simulink model "Main2wheel_simulation"  (R2020b)
settings: Solver=ode4  StartTime=0.0  StopTime=5  FixedStep=0.00001  RelTol=1e-3
libraries: pid_lib x1
settings Model: Creator=Touch  LastModifiedBy=touch

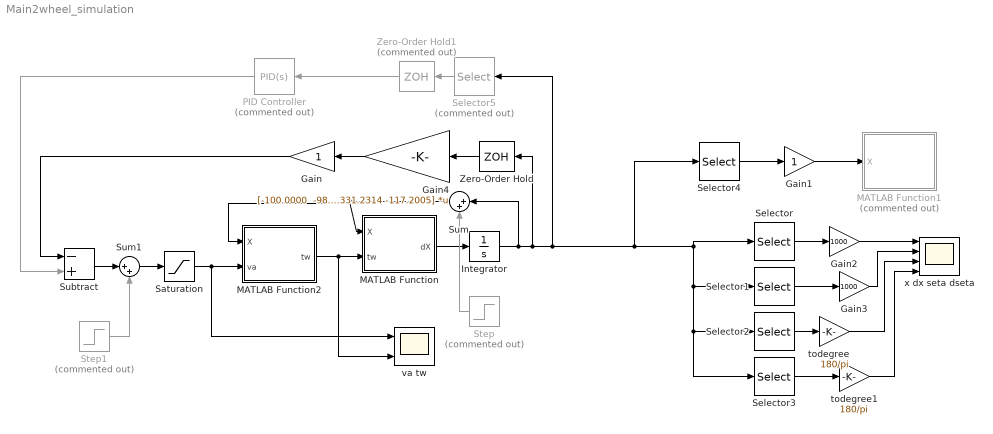
== system Main2wheel_simulation ==
  Gain : Gain
  Gain1 : Gain
  Gain2 : Gain  Gain=1000
  Gain3 : Gain  Gain=1000
  Gain4 : Gain  Gain="[-100.0000  -98.0599 -331.2314 -117.2005]"  Multiplication=Matrix(K*u)
  Integrator : Integrator  InitialCondition=[0;0;0.3;0]  UpperSaturationLimit=[inf;inf;pi/2;inf]  LowerSaturationLimit=[-inf;-inf;-pi/2;-inf]
  MATLAB Function : MATLAB Function  TreatAsAtomicUnit=on
  MATLAB Function1 : MATLAB Function  Commented=on  TreatAsAtomicUnit=on
  MATLAB Function2 : MATLAB Function  TreatAsAtomicUnit=on
  PID Controller : pid_lib/PID Controller  Commented=on  Controller=PID  Form=Parallel  TimeDomain=Continuous-time  UseExternalTs=off  SampleTime=-1  IntegratorMethod=Forward Euler  FilterMethod=Forward Euler  ControllerParametersSource=internal  P=382.730382438672  I=7234.88339162339  D=3.35519935039221  UseFilter=on  N=14917.0518268437  TunerSelectOption=Transfer Function Based (PID Tuner App)  InitialConditionSource=internal  InitialConditionForIntegrator=0  InitialConditionForFilter=0  DifferentiatorICPrevScaledInput=0  ExternalReset=none  TrackingMode=off  Kt=1  LimitOutput=off  SatLimitsSource=internal  UpperSaturationLimit=inf  LowerSaturationLimit=-inf  LinearizeAsGain=on  AntiWindupMode=none  Kb=1  POutMin=[]  POutMax=[]  IOutMin=[]  IOutMax=[]  DOutMin=[]  DOutMax=[]  NOutMin=[]  NOutMax=[]  SumOutMin=[]  SumOutMax=[]  SaturationOutMin=[]  SaturationOutMax=[]  PParamMin=[]  PParamMax=[]  IParamMin=[]  IParamMax=[]  DParamMin=[]  DParamMax=[]  NParamMin=[]  NParamMax=[]  KbParamMin=[]  KbParamMax=[]  KtParamMin=[]  KtParamMax=[]  KbOutMin=[]  KbOutMax=[]  KtOutMin=[]  KtOutMax=[]  IntegratorOutMin=[]  IntegratorOutMax=[]  FilterOutMin=[]  FilterOutMax=[]  SumI1OutMin=[]  SumI1OutMax=[]  SumI2OutMin=[]  SumI2OutMax=[]  SumI3OutMin=[]  SumI3OutMax=[]  SumI4OutMin=[]  SumI4OutMax=[]  SumDOutMin=[]  SumDOutMax=[]  DifferentiatorOutMin=[]  DifferentiatorOutMax=[]  FilterDiffOutCoefMin=[]  FilterDiffOutCoefMax=[]  ReciprocalOutMin=[]  ReciprocalOutMax=[]  SumDenOutMin=[]  SumDenOutMax=[]  SumNumOutMin=[]  SumNumOutMax=[]  DivideOutMin=[]  DivideOutMax=[]  UdiffTsProdOutMin=[]  UdiffTsProdOutMax=[]  NTsProdOutMin=[]  NTsProdOutMax=[]  UintegralTsProdOutMin=[]  UintegralTsProdOutMax=[]  UngainTsProdOutMin=[]  UngainTsProdOutMax=[]  IntegratorContinuousStateAttributes=''  IntegratorStateMustResolveToSignalObject=off  IntegratorRTWStateStorageClass=Auto  FilterContinuousStateAttributes=''  FilterStateMustResolveToSignalObject=off  FilterRTWStateStorageClass=Auto  ParallelPVariant=InternalParameters  IdealPVariant=Disabled  IVariant=InternalParameters  DVariant=InternalParameters  IntegratorVariant=Continuous  SatVariant=Disabled  AWVariant=Passthrough  PCopyVariant=Disabled  TRVariant=Disabled  FdbkBlocksVariant=Forward  IdealPFdbkVariant=Disabled  SatFdbkVariant=Disabled  DerivativeFilterVariant=ContFilter  NVariant=InternalParameters  NCopyVariant=Disabled  FilterICVariant=InternalICsFilter  IntegratorICVariant=InternalICs  ExternalResetVariant=Disabled  TRSumVariant=Passthrough  SumFdbkVariant=Disabled  SumVariant=Sum_PID  TsampFilterVariant=InternalTs  TsampNgainVariant=Passthrough  TsampIntegralVariant=Passthrough  ExternalSaturationOutDataTypeStr=Inherit: Same as second input
  Saturation : Saturate  UpperLimit=24  LowerLimit=-24
  Selector : Selector  InputPortWidth=4  IndexOptions=Index vector (dialog)  Indices=[1]  OutputSizes=1
  Selector1 : Selector  InputPortWidth=4  IndexOptions=Index vector (dialog)  Indices=[2]  OutputSizes=1
  Selector2 : Selector  InputPortWidth=4  IndexOptions=Index vector (dialog)  Indices=[3]  OutputSizes=1
  Selector3 : Selector  InputPortWidth=4  IndexOptions=Index vector (dialog)  Indices=[4]  OutputSizes=1
  Selector4 : Selector  InputPortWidth=4  IndexOptions=Index vector (dialog)  Indices=[1 3]  OutputSizes=1
  Selector5 : Selector  Commented=on  InputPortWidth=4  IndexOptions=Index vector (dialog)  Indices=[3]  OutputSizes=1
  Step : Step  Commented=on  After=[0;0;0.02;0]  SampleTime=4
  Step1 : Step  Commented=on  After=5  SampleTime=.5
  Subtract : Sum  Inputs=-+
  Sum : Sum  Inputs=|++
  Sum1 : Sum  Inputs=|++
  Zero-Order Hold : ZeroOrderHold  SampleTime=0.0055
  Zero-Order Hold1 : ZeroOrderHold  Commented=on  SampleTime=0.0035
  todegree : Gain  Gain=180/pi
  todegree1 : Gain  Gain=180/pi
  va tw : Scope  NumInputPorts=2
  x dx seta dseta : Scope  NumInputPorts=4
  wires:
  Selector/1 -> Gain2/1
  Selector1/1 -> Gain3/1
  Selector3/1 -> todegree1/1
  MATLAB Function/1(dX) -> Integrator/1
  Gain4/1 -> Gain/1
  Selector4/1 -> Gain1/1
  Selector2/1 -> todegree/1
  todegree/1 -> x dx seta dseta/3
  Gain1/1 -> MATLAB Function1/1(X)
  Integrator/1 -> Sum/1, Zero-Order Hold/1, Selector5/1, Selector4/1, Selector/1, Selector3/1, Selector2/1, Selector1/1
  Gain/1 -> Subtract/1
  Gain2/1 -> x dx seta dseta/1
  Gain3/1 -> x dx seta dseta/2
  todegree1/1 -> x dx seta dseta/4
  Zero-Order Hold/1 -> Gain4/1
  PID Controller/1 -> Subtract/2
  Selector5/1 -> Zero-Order Hold1/1
  Zero-Order Hold1/1 -> PID Controller/1
  Saturation/1 -> va tw/1, MATLAB Function2/2(va)
  MATLAB Function2/1(tw) -> va tw/2, MATLAB Function/2(tw)
  Sum/1 -> MATLAB Function2/1(X), MATLAB Function/1(X)
  Step/1 -> Sum/2
  Step1/1 -> Sum1/2
  Subtract/1 -> Sum1/1
  Sum1/1 -> Saturation/1

== matlab function Main2wheel_simulation/MATLAB Function1 ==
  data: X input
function picture(X)
r=0.0335; 
l=.1; 
xw=X(1,1);
setab=X(2,1);

%#codegen
% Define the extrinsic functions

coder.extrinsic('pause')
if ~ishandle(1) %Initialize Figure
     figure(1);
end
clf

pw=[xw r];
pb=[xw+l*sin(setab) l*cos(setab)+r];
line([pw(1) pb(1)],[pw(2) pb(2)],  'LineWidth',3,   'Color',[1 0.4 0.1]);
hold on 
%% Ground
rectangle('Position',[-3.5,0-.1,7,0.1],'FaceColor',[0.6 0.6 0.7])
%% Axis
% grid on
axis([-.3 .3 -.3 .3])
xlabel('X')
ylabel('Y')

end

== matlab function Main2wheel_simulation/MATLAB Function ==
  data: X input; dX output; tw input
function dX = plant(X,tw)

%%model
%%mw=0.3545;
%%r=0.0335; 
%%mb=3-mw;
%%real
mw=5;
r=0.085; 
mb=15;

l=0.03; 
g=9.81; 


xw=X(1,1);
dxw=X(2,1);
setab=X(3,1);
dsetab=X(4,1);
iw=0.5*mw*r^2;
ib=mb*l^2;

ddxw=(mb*l*sin(setab)*dsetab^2-mb^2*l^2*g*cos(setab)*sin(setab)/(mb*l^2+ib)+2*tw*(1/r+mb*l*cos(setab)/(mb*l^2+ib)))/(mb+2*(mw+iw/r^2)-(mb*l*cos(setab))^2/(mb*l^2+ib));
ddsetab=((mb*l*sin(setab))*(g-mb*l*cos(setab)*dsetab^2/(mb+2*(mw+iw/r^2)))-(2*tw/r)*(r+mb*l*cos(setab)/(mb+2*(mw+iw/r^2))))/(ib+mb*l^2-(mb*l*cos(setab))^2/(mb+2*(mw+iw/r^2)));

%%c1=ib+mb*l^2;
%%c2=mw-iw/r^2-mb/2+mb^2*l^2*cos(setab)^2/(2*c1);
%%ddxw=-mb*l*sin(setab)*dsetab^2/(2*c2)+mb^2*g*l^2*sin(setab)*cos(setab)/(2*c1*c2)-(mb*l*cos(setab)/(c1*c2)+1/(r*c2))*tw;
%%ddsetab=mb*l*cos(setab)*ddxw/c1-mb*g*l*sin(setab)/c1+2*tw/c1;

dX=[dxw;ddxw;dsetab;ddsetab];

== matlab function Main2wheel_simulation/MATLAB Function2 ==
  data: X input; tw output; va input
function tw = motor(X,va)

r=0.0335; 

xw=X(1,1);
dxw=X(2,1);
setab=X(3,1);
dsetab=X(4,1);

%% normal motor
%%tw_stall=4.4*9.81*10^-2;
%%vmax=12;
%%tw_0=0.9*9.81*10^-2;
%%dseta_0=100*2*pi/60;
%% real
tw_stall=16;
vmax=24;
tw_0=8;
dseta_0=200*2*pi/60;

k1=tw_stall/vmax;
k2=(k1*vmax-tw_0)/dseta_0;

tw=k1*va-k2*dxw/r+k2*dsetab;
